simulink model "pos_pid_mbd_sl"  (Simulink 8.7)
settings: Solver=FixedStepDiscrete  StartTime=0.0  StopTime=tfinal  FixedStep=ts  RelTol=1e-3
values from neighbouring files (symbols this model uses):
  dist = 2    [pos_pid_mbd.m]
  Kd = -((p1+p2+p3)*T + 1)/K    [pos_pid_mbd.m]
  Ki = -p1*p2*p3*T/K    [pos_pid_mbd.m]
  Kp = (p1*p2 + p2*p3 + p3*p1)*T/K    [pos_pid_mbd.m]
  r = 60    [pos_pid_mbd.m]
  r_cyc = 4    [pos_pid_mbd.m]
undefined symbols (not defined in the file or in its folder): denpd, DiscIntNeverNeededParam, numpd, ts
libraries: arduinolib x3, simulink x2
settings Model: Creator=hirata  LastModifiedBy=morita  SimulationMode=external  ExtModeTrigDuration=2
settings DataIOCC: SignalLoggingSaveFormat=ModelDataLogs
settings OptimizationCC: ExpressionDepthLimit=2147483647  OptimizeModelRefInitCode=on  LifeSpan=1  MaxStackSize=64
settings DebuggingCC: SolverPrmCheckMsg=warning  FcnCallInpInsideContextMsg=UseLocalSettings  StateNameClashWarn=warning
settings HardwareCC: ProdBitPerInt=16  ProdBitPerPointer=16  ProdIntDivRoundTo=Zero  ProdEndianess=LittleEndian  ProdWordSize=8  ProdHWDeviceType=Atmel->AVR  UseEmbeddedCoderFeatures=off  UseSimulinkCoderFeatures=off
settings RTWCC: SystemTargetFile=ert.tlc  HardwareBoard=Arduino Mega 2560  TLCOptions=-aInlineSetEventsForThisBaseRateFcn=TLC_FALSE -aSuppressMultiTaskScheduler=TLC_FALSE  TemplateMakefile=ert_default_tmf  Description=Embedded Coder  GenerateReport=on  Toolchain=Arduino AVR v1.6.1  BuildConfiguration=Faster Runs  IncludeHyperlinkInReport=on  LaunchReport=on  GenerateTraceInfo=on  GenerateTraceReport=on  GenerateTraceReportSl=on  GenerateTraceReportSf=on  GenerateTraceReportEml=on
settings MATStruct: className=codertarget.tools.BuildHook  argsTopModelOnly=[]  excludedModels=[]  includeReferencedModels=on  includeTopModel=on  enabled=on  UseCoderTarget=[1]  TargetHardware=Arduino Mega 2560  RTOS=Baremetal  Scheduler_interrupt_source=[0.0]  DataVersion=2016.02  Baudrate=115200  COMPort=codertarget.arduinobase.internal.getExternalModeMexArgs('Serial')  Verbose=[0]  IPAddress=codertarget.arduinobase.internal.getExternalModeMexArgs('Ethernet')  Port=17725  Configuration=Serial  BuildAction=Build, load and run  Set_host_COM_port=Automatically  COM_port_number=1  Enable_overrun_detection=[0.0]  Digital_output_to_set_on_overrun=13  Analog_input_reference_voltage=[0.0]  Serial0_baud_rate=9600  Serial1_baud_rate=9600  Serial2_baud_rate=9600  Serial3_baud_rate=9600  SPI_clock_out_frequency=4000  SPI_mode=Mode 0 - Clock Polarity 0, Clock Phase 0  SPI_bitorder=MSB first  Disable_DHCP_Ethernet=[0.0]  Local_ip_address=192.168.0.20  Local_mac_address=DE:AD:BE:EF:FE:ED  Disable_DHCP_Wifi=[0.0]  Wifi_ip_address=192.168.1.20  Wifi_SSID=yourNetwork  Set_Wifi_Encryption=None  Wifi_WEP_key=D0D0DEADF00DABBADEAFBEADED  Wifi_WEP_key_index=0  Wifi_WPA_password=secretPassword
settings CodeAppCC: ForceParamTrailComments=on  IgnoreCustomStorageClasses=off  OperatorAnnotations=on  SimulinkDataObjDesc=on  SFDataObjDesc=on  MATLABFcnDesc=on  InsertBlockDesc=on  MATLABSourceComments=on
settings ERTTargetCC: MultiwordLength=2048  SupportContinuousTime=on  SupportNonInlinedSFcns=on  SupportVariableSizeSignals=on

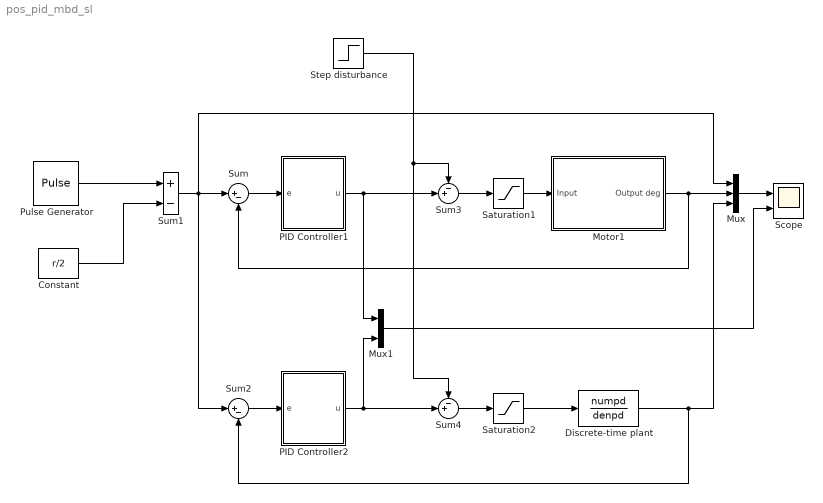
== system pos_pid_mbd_sl ==
  Constant : Constant  Value=r/2
  Discrete-time plant : DiscreteTransferFcn  Numerator=numpd  Denominator=denpd
  Motor1 : Subsystem
  Mux : Mux  Inputs=3
  Mux1 : Mux  Inputs=2
  PID Controller1 : Subsystem
  PID Controller2 : Subsystem
  Pulse Generator : DiscretePulseGenerator  PulseType=Time based  Amplitude=r  Period=r_cyc  PulseWidth=50
  Saturation1 : Saturate  UpperLimit=5  LowerLimit=-5
  Saturation2 : Saturate  UpperLimit=5  LowerLimit=-5
  Scope : Scope  NumInputPorts=2
  Step disturbance : Step  Time=r_cyc/4  After=dist  SampleTime=ts
  Sum : Sum  Inputs=|+-
  Sum1 : Sum  Inputs=+-
  Sum2 : Sum  Inputs=|+-
  Sum3 : Sum  Inputs=-+|
  Sum4 : Sum  Inputs=-+|
  wires:
  PID Controller1/1(u) -> Mux1/1, Sum3/2
  Sum/1 -> PID Controller1/1(e)
  Sum1/1 -> Sum/1, Mux/1, Sum2/1
  Motor1/1(Output deg) -> Sum/2, Mux/2
  Pulse Generator/1 -> Sum1/1
  Constant/1 -> Sum1/2
  Mux/1 -> Scope/1
  PID Controller2/1(u) -> Mux1/2, Sum4/2
  Sum2/1 -> PID Controller2/1(e)
  Mux1/1 -> Scope/2
  Discrete-time plant/1 -> Sum2/2, Mux/3
  Step disturbance/1 -> Sum4/1, Sum3/1
  Sum3/1 -> Saturation1/1
  Sum4/1 -> Saturation2/1
  Saturation1/1 -> Motor1/1(Input)
  Saturation2/1 -> Discrete-time plant/1

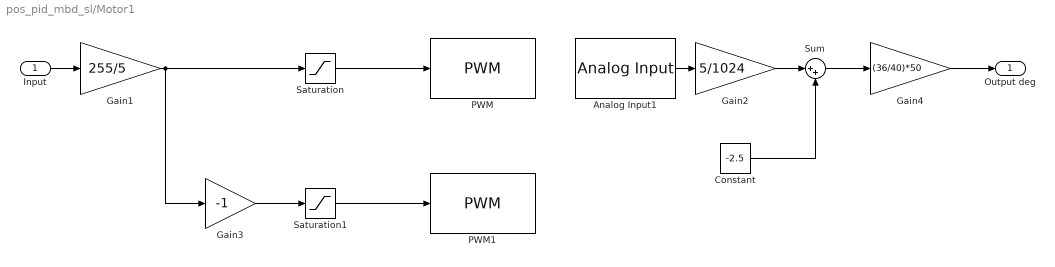
== system pos_pid_mbd_sl/Motor1 ==
  Input : Inport
  Analog Input1 : arduinolib/Analog Input  pinNumber=0  sampleTime=ts  blockPlatform=arduino
  Constant : Constant  Value=-2.5
  Gain1 : Gain  Gain=255/5
  Gain2 : Gain  Gain=5/1024
  Gain3 : Gain  Gain=-1
  Gain4 : Gain  Gain=(36/40)*50
  PWM : arduinolib/PWM  pinNumber=3  blockPlatform=arduino
  PWM1 : arduinolib/PWM  pinNumber=5  blockPlatform=arduino
  Saturation : Saturate  UpperLimit=255  LowerLimit=0
  Saturation1 : Saturate  UpperLimit=255  LowerLimit=0
  Sum : Sum  Inputs=|++
  Output deg : Outport
  wires:
  Input/1 -> Gain1/1
  Analog Input1/1 -> Gain2/1
  Saturation/1 -> PWM/1
  Gain1/1 -> Gain3/1, Saturation/1
  Saturation1/1 -> PWM1/1
  Gain4/1 -> Output deg/1
  Gain2/1 -> Sum/1
  Sum/1 -> Gain4/1
  Constant/1 -> Sum/2
  Gain3/1 -> Saturation1/1

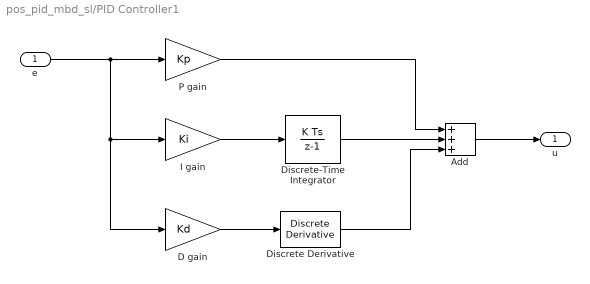
== system pos_pid_mbd_sl/PID Controller1 ==
  e : Inport
  Add : Sum  Inputs=+++
  D gain : Gain  Gain=Kd
  Discrete Derivative : simulink/Discrete/Discrete Derivative  gainval=1.0  ICPrevScaledInput=0.0  InputProcessing=Inherited  OutMin=[]  OutMax=[]  OutDataType=fixdt(1, 16)  OutScaling=2^-10  DoSatur=off
  Discrete-Time Integrator : DiscreteIntegrator  SampleTime=ts  ICPrevOutput=DiscIntNeverNeededParam  ICPrevScaledInput=DiscIntNeverNeededParam
  I gain : Gain  Gain=Ki
  P gain : Gain  Gain=Kp
  u : Outport
  wires:
  I gain/1 -> Discrete-Time Integrator/1
  P gain/1 -> Add/1
  Discrete-Time Integrator/1 -> Add/2
  e/1 -> P gain/1, I gain/1, D gain/1
  Add/1 -> u/1
  Discrete Derivative/1 -> Add/3
  D gain/1 -> Discrete Derivative/1

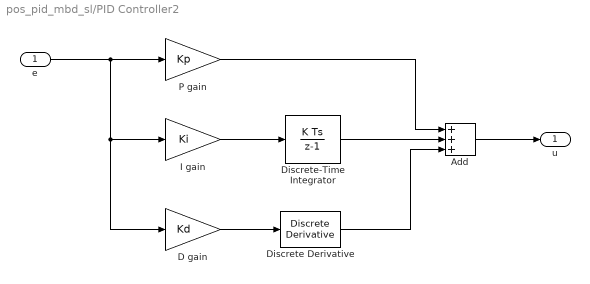
== system pos_pid_mbd_sl/PID Controller2 ==
  e : Inport
  Add : Sum  Inputs=+++
  D gain : Gain  Gain=Kd
  Discrete Derivative : simulink/Discrete/Discrete Derivative  gainval=1.0  ICPrevScaledInput=0.0  InputProcessing=Inherited  OutMin=[]  OutMax=[]  OutDataType=fixdt(1, 16)  OutScaling=2^-10  DoSatur=off
  Discrete-Time Integrator : DiscreteIntegrator  SampleTime=ts  ICPrevOutput=DiscIntNeverNeededParam  ICPrevScaledInput=DiscIntNeverNeededParam
  I gain : Gain  Gain=Ki
  P gain : Gain  Gain=Kp
  u : Outport
  wires:
  I gain/1 -> Discrete-Time Integrator/1
  P gain/1 -> Add/1
  Discrete-Time Integrator/1 -> Add/2
  e/1 -> P gain/1, I gain/1, D gain/1
  Add/1 -> u/1
  Discrete Derivative/1 -> Add/3
  D gain/1 -> Discrete Derivative/1
